simulink library "ava"  (Simulink 8.1)
settings: Solver=ode1  StartTime=0.0  StopTime=Inf  FixedStep=0.001  RelTol=1e-3
PostLoadFcn:
  | , if any(exist('dsrtsu_mdlpostloadfcn', 'file') == [2, 3, 6]), try dsrtsu_mdlpostloadfcn('Execute', bdroot); catch fprintf('Error in PostLoadFcn (dsrtsu_mdlpostloadfcn) for model "%s":\n %s\n', bdroot, lasterr); end, end,
undefined symbols (not defined in the file or in its folder): C_TICK_TIME_S, FALSE, TRUE
libraries: hcu_lib x1
settings Model: DSRTSU_INTERNAL_RTI_VER=450  DSRTSU_INTERNAL_RTI_TYPE=rti1401  RTICANMMDATA=struct('GeneralSetupData',struct('modelroot','D:\ELN150201\Phase3\branches\ACC_Experiments\AdasDragon\software\sw_development\arch\app\jud','generalsettings',struct('filesettings',struct('destfolder',struct('Name','RTICANMM_FILES','Check',1),'buildfolder',struct('Name','.','Check',1),'AbsDestfolder',struct('Name','D:\ELN150201\Phase3\branches\ACC_Experiments\AdasDragon\software\sw_development\arch\app\jud\RTICANMM_FILES'),'AbsBuildfolder',struct('Name','D:\ELN150201\Phase3\branches\ACC_Experiments\AdasDragon\software\sw_development\arch\app\jud'))),'options',struct('addpaths',1,'rmpaths',1,'addtrcexclusion',logical(1),'cannavigator',struct('checkmonitoring',0),'show_usrtrc',0,'use_usrtrc',0),'advanced',struct('options',[1 1 1 1 1 1 1 1 1 1 1 1 1 1 1 1 1 1 1 1 1 1 1 1 1 1 1 1 1 1 1 1 1 1 1 1 1 1 1 1 1 1 1 1 1 1 1 1 1 1 1 1 1 1 1 1 1 1 1 1 1 1 1 1 1 1 1 1 1 1 1 1 1 1 1 1 1 1 1 1 1 1 1 1 1 1 1 1 1 1 1 1 1 1 1 1 1 1 1 1]),'MPSetup',{{}},'modelname','ava','block','ava'))  DSRTSU_INTERNAL_RTIFPGA=40  Creator=tescamilla  LastModifiedBy=AT015555

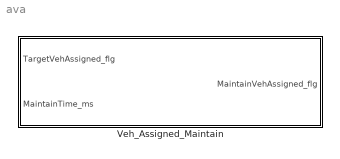
== system ava ==
  Veh_Assigned_Maintain : Subsystem

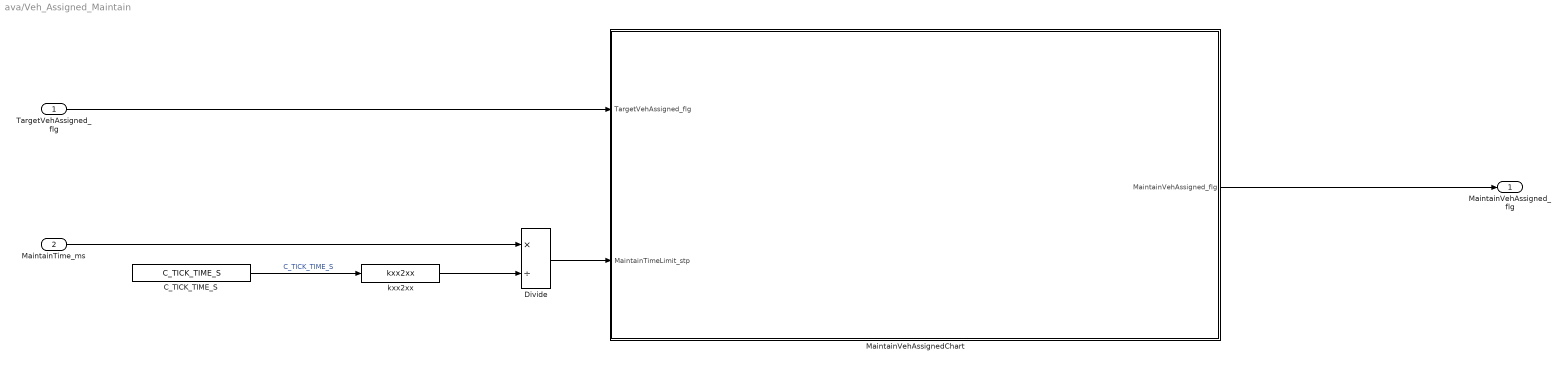
== system ava/Veh_Assigned_Maintain ==
  TargetVehAssigned_flg : Inport
  MaintainTime_ms : Inport  Port=2
  C_TICK_TIME_S : Constant  Value=C_TICK_TIME_S
  Divide : Product  Inputs=*/
  MaintainVehAssignedChart : Stateflow chart  TreatAsAtomicUnit=on
  kxx2xx : hcu_lib/kxx2xx
  MaintainVehAssigned_flg : Outport
  wires:
  MaintainTime_ms/1 -> Divide/1
  kxx2xx/1 -> Divide/2
  Divide/1 -> MaintainVehAssignedChart/2(MaintainTimeLimit_stp)
  C_TICK_TIME_S/1 -> kxx2xx/1  "C_TICK_TIME_S"
  TargetVehAssigned_flg/1 -> MaintainVehAssignedChart/1(TargetVehAssigned_flg)
  MaintainVehAssignedChart/1(MaintainVehAssigned_flg) -> MaintainVehAssigned_flg/1

== stateflow chart Veh_Assigned_Maintain/MaintainVehAssignedChart ==
  state VEH_NOT_ASSIGNED
    en:
    MaintainVehAssigned_flg = FALSE;
  state VEH_ASSIGNED
    en:
    MaintainVehAssigned_flg = TRUE;
  state MAINTAIN
    en:
    MaintainTimeLocal_stp = 0;
    du:
    MaintainTimeLocal_stp=MaintainTimeLocal_stp+1;
  (default) -> VEH_NOT_ASSIGNED
  (junction 12) -> VEH_NOT_ASSIGNED : [MaintainTimeLocal_stp>MaintainTimeLimit_stp...
      | && TargetVehAssigned_flg ==FALSE]
  MAINTAIN -> (junction 12) [order 2]
  VEH_NOT_ASSIGNED -> (junction 13)
  VEH_ASSIGNED -> MAINTAIN : [TargetVehAssigned_flg==FALSE]
  (junction 13) -> VEH_ASSIGNED : [TargetVehAssigned_flg==TRUE]
  MAINTAIN -> VEH_ASSIGNED [order 1] : [TargetVehAssigned_flg ==TRUE]
  data: MaintainVehAssigned_flg output boolean; TargetVehAssigned_flg input boolean; FALSE parameter double; TRUE parameter double; MaintainTimeLocal_stp local single; MaintainTimeLimit_stp input single
